simulink model "TargetDetection"  (R2016b)
settings: Solver=VariableStepAuto  StartTime=0.0  StopTime=10  RelTol=1e-3
undefined symbols (not defined in the file or in its folder): designMultirateFIR, magnitude, physconst
libraries: phasedenvlib x6, phaseddetectlib x2, phasedtxrxlib x2, simulink x1, dspmlti4 x1, phasedwavlib x1, dspsigops x1
settings Model: Creator=CHAITRA  LastModifiedBy=CHAITRA

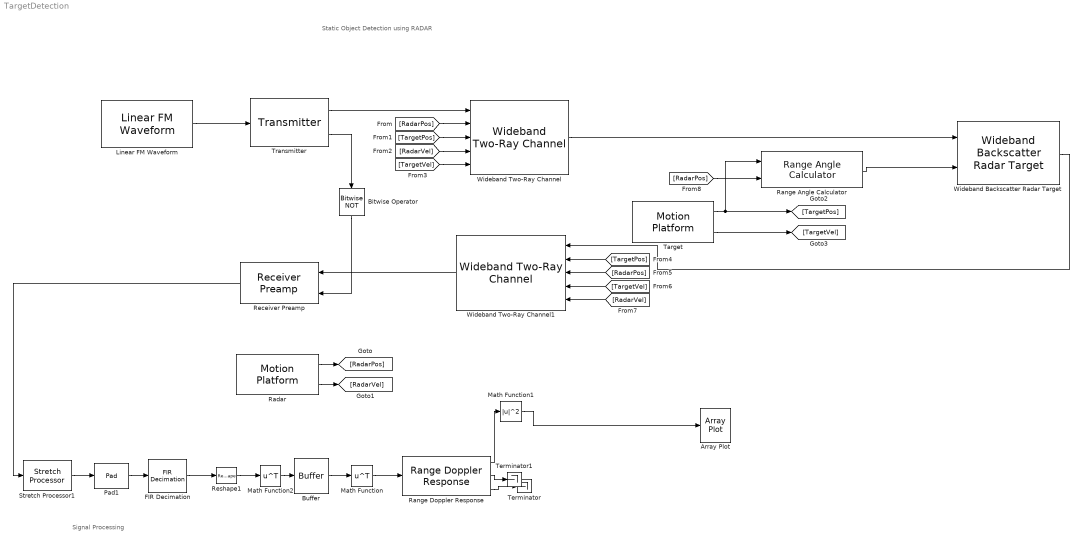
== system TargetDetection ==
  note: Static Object Detection using RADAR
  note: Signal Processing
  Array Plot : ArrayPlot
  Bitwise Operator : simulink/Logic and Bit Operations/Bitwise Operator  logicop=NOT  UseBitMask=off  BitMask=bin2dec('11011001')  BitMaskRealWorld=Stored Integer
  Buffer : Buffer  N=5  TreatMby1Signals=One channel  OutputFrames=off
  FIR Decimation : dspmlti4/FIR Decimation  FilterSource=Auto  h=designMultirateFIR(1,2)  D=4  filtStruct=Direct form  FilterObject=FDECIM  InputProcessing=Columns as channels (frame based)  framing=Enforce single-rate processing  inputOffset=0  outputBufInitCond=0  roundingMode=Floor  overflowMode=off  firstCoeffDataTypeStr=Inherit: Same word length as input  firstCoeffMin=[]  firstCoeffMax=[]  firstCoeffLastDataTypeStr=Inherit: Same word length as input  outputDataTypeStr=Inherit: Same as accumulator  outputMin=[]  outputMax=[]  outputLastDataTypeStr=Inherit: Same as accumulator
  Linear FM Waveform : phasedwavlib/Linear FM Waveform  SampleRate=200e6  DurationSpecification=Pulse width  PulseWidth=1e-8  DutyCycle=0.5  PRF=1e7  PRFSelectionInputPort=off  SweepBandwidth=100e6  SweepDirection=Up  SweepInterval=Positive  Envelope=Rectangular  OutputFormat=Pulses  NumSamples=100  NumPulses=1  SimulateUsing=Interpreted execution
  Math Function : Math  Operator=transpose  SaturateOnIntegerOverflow=on
  Math Function1 : Math  Operator=magnitude^2  SaturateOnIntegerOverflow=on
  Math Function2 : Math  Operator=transpose  SaturateOnIntegerOverflow=on
  Pad1 : dspsigops/Pad  padAlong=Columns  dimsToPad=1  valSrc=Specify via dialog  padVal=0  spec=Output size  padNumOutRowsSpecMethod=User-specified  numOutRows=20  padNumOutColsSpecMethod=User-specified  numOutCols=1  isVarDimsMode=off  padBeginning=0  padEnd=0  outSizeMode=User-specified  outSize=1  padSigAt=End  trunc_flag=None  roundingMode=Floor  overflowMode=off  truncOrWrapMode=Truncate  wrap_flag=None
  "Radar " : phasedenvlib/Motion Platform  MotionModel=Velocity  InitialPosition=[ 0; 0; 0 ]  InitialVelocity=[ 0; 0; 0 ]  VelocitySource=Property  Velocity=[0;0;0]  AccelerationSource=Property  Acceleration=[0;0;0]  InitialOrientationAxes=eye( 3 )  OrientationAxesOutputPort=off  ElapsedTimeSource=Auto  SampleRateFromInputCheckbox=on  SampleRate=1e6  SimulateUsing=Interpreted execution
  Range Angle Calculator : phasedenvlib/Range Angle Calculator  Model=Free space  ReferencePositionSource=Input port  ReferencePosition=[ 0; 0; 0 ]  ReferenceAxesSource=Property  ReferenceAxes=eye( 3 )  Output=Angle  SimulateUsing=Interpreted execution
  Range Doppler Response : phaseddetectlib/Range Doppler Response  RangeMethod=FFT  PropagationSpeed=3e8  SampleRateFromInputCheckbox=on  SampleRate=1e6  SweepSlope=1e16  DechirpInput=off  RangeFFTLengthSource=Auto  RangeFFTLength=1024  RangeWindow=Taylor  RangeSidelobeAttenuation=30  CustomRangeWindow=@hamming  MaximumNumInputSamplesSource=Auto  MaximumNumInputSamples=100  DopplerFFTLengthSource=Property  DopplerFFTLength=32  DopplerWindow=Taylor  DopplerSidelobeAttenuation=30  CustomDopplerWindow=@hamming  DopplerOutput=Frequency  OperatingFrequency=800e6  SimulateUsing=Interpreted execution
  Receiver Preamp : phasedtxrxlib/Receiver Preamp  Gain=20  LossFactor=0  NoiseMethod=Noise temperature  NoiseFigure=0  ReferenceTemperature=290  SampleRateFromInputCheckbox=on  SampleRate=1e6  NoisePower=0  EnableInputPort=on  PhaseNoiseInputPort=off  SeedSource=Property  Seed=randi(65535,1)  SimulateUsing=Interpreted execution
  Reshape1 : Reshape
  Stretch Processor1 : phaseddetectlib/Stretch Processor  PulseWidth=1e-8  PRF=1e7  SweepSlope=1e16  SweepInterval=Positive  PropagationSpeed=3e8  ReferenceRange=7  RangeSpan=1  SimulateUsing=Interpreted execution
  "Target " : phasedenvlib/Motion Platform  MotionModel=Velocity  InitialPosition=[ 7; 0; 0 ]  InitialVelocity=[ 0; 0; 0 ]  VelocitySource=Property  Velocity=[0;0;0]  AccelerationSource=Property  Acceleration=[0;0;0]  InitialOrientationAxes=eye( 3 )  OrientationAxesOutputPort=off  ElapsedTimeSource=Auto  SampleRateFromInputCheckbox=on  SampleRate=1e6  SimulateUsing=Interpreted execution
  Terminator : Terminator
  Terminator1 : Terminator
  Transmitter : phasedtxrxlib/Transmitter  PeakPower=1e-3  Gain=20  LossFactor=0  InUseOutputPort=on  CoherentOnTransmit=on  PhaseNoiseOutputPort=off  SeedSource=Property  Seed=randi(65535,1)  SimulateUsing=Interpreted execution
  Wideband Backscatter Radar Target : phasedenvlib/Wideband Backscatter Radar Target  EnablePolarization=off  FrequencyVector=[ 0, 1e20 ]  AzimuthAngles=-180:20:180  ElevationAngles=0  RCSPattern=zeros(1,19)  ShhPattern=ones(181,361)  ShvPattern=ones(181,361)  SvvPattern=ones(181,361)  Model=Nonfluctuating  PropagationSpeed=physconst( 'LightSpeed' )  OperatingFrequency=800e6  SampleRateFromInputCheckbox=on  SampleRate=1e6  NumSubbands=20  SeedSource=Property  Seed=randi(65535,1)  SimulateUsing=Interpreted execution
  Wideband Two-Ray Channel : phasedenvlib/Wideband Two-Ray Channel  PropagationSpeed=physconst( 'LightSpeed' )  OperatingFrequency=3e8  NumSubbands=20  SpecifyAtmosphere=off  Temperature=15  DryAirPressure=101325  WaterVapourDensity=7.5  LiquidWaterDensity=0  RainRate=0  SampleRateFromInputCheckbox=on  SampleRate=1e6  GroundReflectionCoefficient=-1  GroundRelativePermittivity=15  CombinedRaysOutput=on  MaximumDistanceSource=Property  MaximumDistance=15  MaximumNumInputSamplesSource=Auto  MaximumNumInputSamples=1000  SimulateUsing=Interpreted execution
  Wideband Two-Ray Channel1 : phasedenvlib/Wideband Two-Ray Channel  PropagationSpeed=physconst( 'LightSpeed' )  OperatingFrequency=3e8  NumSubbands=20  SpecifyAtmosphere=off  Temperature=15  DryAirPressure=101325  WaterVapourDensity=7.5  LiquidWaterDensity=0  RainRate=0  SampleRateFromInputCheckbox=on  SampleRate=1e6  GroundReflectionCoefficient=-1  GroundRelativePermittivity=15  CombinedRaysOutput=on  MaximumDistanceSource=Property  MaximumDistance=15  MaximumNumInputSamplesSource=Auto  MaximumNumInputSamples=1000  SimulateUsing=Interpreted execution
  wires:
  Bitwise Operator/1 -> Receiver Preamp/2
  "Radar "/1 -> [RadarPos]
  "Radar "/2 -> [RadarVel]
  Transmitter/2 -> Bitwise Operator/1
  Transmitter/1 -> Wideband Two-Ray Channel/1
  [TargetVel] -> Wideband Two-Ray Channel/5
  [RadarVel] -> Wideband Two-Ray Channel/4
  [TargetPos] -> Wideband Two-Ray Channel/3
  [RadarPos] -> Wideband Two-Ray Channel/2
  Wideband Two-Ray Channel1/1 -> Receiver Preamp/1
  [TargetPos] -> Wideband Two-Ray Channel1/2
  [RadarPos] -> Wideband Two-Ray Channel1/3
  [TargetVel] -> Wideband Two-Ray Channel1/4
  [RadarVel] -> Wideband Two-Ray Channel1/5
  Wideband Two-Ray Channel/1 -> Wideband Backscatter Radar Target/1
  Range Angle Calculator/1 -> Wideband Backscatter Radar Target/2
  [RadarPos] -> Range Angle Calculator/2
  "Target "/2 -> [TargetVel]
  "Target "/1 -> Range Angle Calculator/1, [TargetPos]
  Wideband Backscatter Radar Target/1 -> Wideband Two-Ray Channel1/1
  Receiver Preamp/1 -> Stretch Processor1/1
  Reshape1/1 -> Math Function2/1
  FIR Decimation/1 -> Reshape1/1
  Stretch Processor1/1 -> Pad1/1
  Pad1/1 -> FIR Decimation/1
  Buffer/1 -> Math Function/1
  Math Function2/1 -> Buffer/1
  Range Doppler Response/3 -> Terminator/1
  Range Doppler Response/2 -> Terminator1/1
  Linear FM Waveform/1 -> Transmitter/1
  Range Doppler Response/1 -> Math Function1/1
  Math Function1/1 -> Array Plot/1
  Math Function/1 -> Range Doppler Response/1
